simulink model "picture_prototype"  (R2022a)
settings: Solver=FixedStepAuto  StartTime=0.0  StopTime=80000  RelTol=1e-3
undefined symbols (not defined in the file): area_air, cp_air, HC_min, HC_nom, rho_air, sigbuilder_block, Ts, vel_air_nom
libraries: fl_lib x61, nesl_utility x24, SimscapeFluids_lib x5, ee_lib x4, sdl_lib x2
(part 2 of 2)

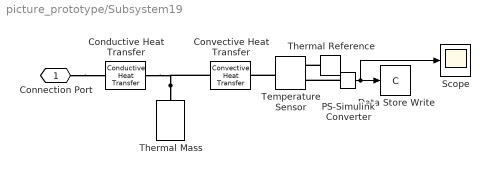
== system picture_prototype/Subsystem19 ==
  Conductive Heat Transfer : fl_lib/Thermal/Thermal Elements/Conductive Heat Transfer  area=1e-4 m^2  thickness=0.1 m  th_cond=401 W/(K*m)  T_specify=off  T_priority=None  T=0 K  T_nominal_specify=off  T_nominal_unit=K  T_nominal_value=1  Q_specify=off  Q_priority=None  Q=0 W  Q_nominal_specify=off  Q_nominal_unit=W  Q_nominal_value=1
      settings: SourceProductBaseCode=PW,SS,VE
  Convective Heat Transfer : fl_lib/Thermal/Thermal Elements/Convective Heat Transfer  area=1e-4 m^2  heat_tr_coeff=20 W/(K*m^2)  T_specify=off  T_priority=None  T=0 K  T_nominal_specify=off  T_nominal_unit=K  T_nominal_value=1  Q_specify=off  Q_priority=None  Q=0 W  Q_nominal_specify=off  Q_nominal_unit=W  Q_nominal_value=1
      settings: SourceProductBaseCode=PW,SS,VE
  Data Store Write : DataStoreWrite  DataStoreName=C  IndexOptions=Index vector (dialog)  Indices=1  OutputSizes=1
  PS-Simulink Converter : nesl_utility/PS-Simulink Converter  PhysicalDomain=network_engine_domain  SubClassName=ps_output  LeftPortType=input  RightPortType=output  PseudoPeriodic=off  Frequencies=[]  VectorFormat=inherit  Unit=inherit  AffineConversion=off
      settings: SourceProductBaseCode=SS,PW,VE
  Scope : Scope
  Temperature Sensor : fl_lib/Thermal/Thermal Sensors/Temperature Sensor
      settings: SourceProductBaseCode=PW,SS,VE
  Thermal Mass : fl_lib/Thermal/Thermal Elements/Thermal Mass  mass=1 kg  sp_heat=447 J/(K*kg)  T_specify=off  T_priority=High  T=300 K  T_nominal_specify=off  T_nominal_unit=K  T_nominal_value=1  Q_specify=off  Q_priority=None  Q=0 W  Q_nominal_specify=off  Q_nominal_unit=W  Q_nominal_value=1
      settings: SourceProductBaseCode=PW,SS,VE
  Thermal Reference : fl_lib/Thermal/Thermal Elements/Thermal Reference
      settings: SourceProductBaseCode=PW,SS,VE
  Connection Port : PMIOPort  Side=Left
  wires:
  PS-Simulink Converter/1 -> Data Store Write/1, Scope/1
  connections:
  Connection Port/RConn1 -- Conductive Heat Transfer/LConn1
  Thermal Mass/LConn1 -- Conductive Heat Transfer/RConn1 -- Convective Heat Transfer/LConn1
  Temperature Sensor/LConn1 -- Convective Heat Transfer/RConn1
  Thermal Reference/LConn1 -- Temperature Sensor/RConn1
  PS-Simulink Converter/LConn1 -- Temperature Sensor/RConn2

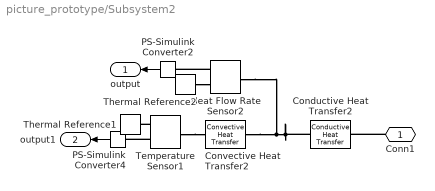
== system picture_prototype/Subsystem2 ==
  Conductive Heat Transfer2 : fl_lib/Thermal/Thermal Elements/Conductive Heat Transfer  area=1e-4 m^2  thickness=0.1 m  th_cond=401 W/(K*m)  T_specify=off  T_priority=None  T=0 K  T_nominal_specify=off  T_nominal_unit=K  T_nominal_value=1  Q_specify=off  Q_priority=None  Q=0 W  Q_nominal_specify=off  Q_nominal_unit=W  Q_nominal_value=1
      settings: SourceProductBaseCode=PW,SS,VE
  Convective Heat Transfer2 : fl_lib/Thermal/Thermal Elements/Convective Heat Transfer  area=1e-4 m^2  heat_tr_coeff=20 W/(K*m^2)  T_specify=off  T_priority=None  T=0 K  T_nominal_specify=off  T_nominal_unit=K  T_nominal_value=1  Q_specify=off  Q_priority=None  Q=0 W  Q_nominal_specify=off  Q_nominal_unit=W  Q_nominal_value=1
      settings: SourceProductBaseCode=PW,SS,VE
  Heat Flow Rate Sensor2 : fl_lib/Thermal/Thermal Sensors/Heat Flow Rate Sensor
      settings: SourceProductBaseCode=PW,SS,VE
  PS-Simulink Converter2 : nesl_utility/PS-Simulink Converter  PhysicalDomain=network_engine_domain  SubClassName=ps_output  LeftPortType=input  RightPortType=output  PseudoPeriodic=off  Frequencies=[]  VectorFormat=inherit  Unit=inherit  AffineConversion=off
      settings: SourceProductBaseCode=SS,PW,VE
  PS-Simulink Converter4 : nesl_utility/PS-Simulink Converter  PhysicalDomain=network_engine_domain  SubClassName=ps_output  LeftPortType=input  RightPortType=output  PseudoPeriodic=off  Frequencies=[]  VectorFormat=inherit  Unit=inherit  AffineConversion=off
      settings: SourceProductBaseCode=SS,PW,VE
  Temperature Sensor1 : fl_lib/Thermal/Thermal Sensors/Temperature Sensor
      settings: SourceProductBaseCode=PW,SS,VE
  Thermal Reference1 : fl_lib/Thermal/Thermal Elements/Thermal Reference
      settings: SourceProductBaseCode=PW,SS,VE
  Thermal Reference2 : fl_lib/Thermal/Thermal Elements/Thermal Reference
      settings: SourceProductBaseCode=PW,SS,VE
  Conn1 : PMIOPort  Side=Left
  output : Outport
  output1 : Outport  Port=2
  wires:
  PS-Simulink Converter2/1 -> output/1
  PS-Simulink Converter4/1 -> output1/1
  connections:
  Temperature Sensor1/RConn2 -- PS-Simulink Converter4/LConn1
  Thermal Reference2/LConn1 -- Heat Flow Rate Sensor2/RConn2
  Temperature Sensor1/RConn1 -- Thermal Reference1/LConn1
  Temperature Sensor1/LConn1 -- Convective Heat Transfer2/RConn1
  Heat Flow Rate Sensor2/RConn1 -- PS-Simulink Converter2/LConn1
  Conn1/RConn1 -- Conductive Heat Transfer2/LConn1
  Convective Heat Transfer2/LConn1 -- Conductive Heat Transfer2/RConn1 -- Heat Flow Rate Sensor2/LConn1

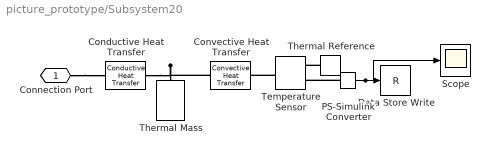
== system picture_prototype/Subsystem20 ==
  Conductive Heat Transfer : fl_lib/Thermal/Thermal Elements/Conductive Heat Transfer  area=1e-4 m^2  thickness=0.1 m  th_cond=401 W/(K*m)  T_specify=off  T_priority=None  T=0 K  T_nominal_specify=off  T_nominal_unit=K  T_nominal_value=1  Q_specify=off  Q_priority=None  Q=0 W  Q_nominal_specify=off  Q_nominal_unit=W  Q_nominal_value=1
      settings: SourceProductBaseCode=PW,SS,VE
  Convective Heat Transfer : fl_lib/Thermal/Thermal Elements/Convective Heat Transfer  area=1e-4 m^2  heat_tr_coeff=20 W/(K*m^2)  T_specify=off  T_priority=None  T=0 K  T_nominal_specify=off  T_nominal_unit=K  T_nominal_value=1  Q_specify=off  Q_priority=None  Q=0 W  Q_nominal_specify=off  Q_nominal_unit=W  Q_nominal_value=1
      settings: SourceProductBaseCode=PW,SS,VE
  Data Store Write : DataStoreWrite  DataStoreName=R  IndexOptions=Index vector (dialog)  Indices=1  OutputSizes=1
  PS-Simulink Converter : nesl_utility/PS-Simulink Converter  PhysicalDomain=network_engine_domain  SubClassName=ps_output  LeftPortType=input  RightPortType=output  PseudoPeriodic=off  Frequencies=[]  VectorFormat=inherit  Unit=inherit  AffineConversion=off
      settings: SourceProductBaseCode=SS,PW,VE
  Scope : Scope
  Temperature Sensor : fl_lib/Thermal/Thermal Sensors/Temperature Sensor
      settings: SourceProductBaseCode=PW,SS,VE
  Thermal Mass : fl_lib/Thermal/Thermal Elements/Thermal Mass  mass=1 kg  sp_heat=447 J/(K*kg)  T_specify=off  T_priority=High  T=300 K  T_nominal_specify=off  T_nominal_unit=K  T_nominal_value=1  Q_specify=off  Q_priority=None  Q=0 W  Q_nominal_specify=off  Q_nominal_unit=W  Q_nominal_value=1
      settings: SourceProductBaseCode=PW,SS,VE
  Thermal Reference : fl_lib/Thermal/Thermal Elements/Thermal Reference
      settings: SourceProductBaseCode=PW,SS,VE
  Connection Port : PMIOPort  Side=Left
  wires:
  PS-Simulink Converter/1 -> Data Store Write/1, Scope/1
  connections:
  Connection Port/RConn1 -- Conductive Heat Transfer/LConn1
  Thermal Mass/LConn1 -- Conductive Heat Transfer/RConn1 -- Convective Heat Transfer/LConn1
  Temperature Sensor/LConn1 -- Convective Heat Transfer/RConn1
  Thermal Reference/LConn1 -- Temperature Sensor/RConn1
  PS-Simulink Converter/LConn1 -- Temperature Sensor/RConn2

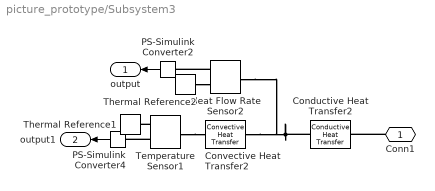
== system picture_prototype/Subsystem3 ==
  Conductive Heat Transfer2 : fl_lib/Thermal/Thermal Elements/Conductive Heat Transfer  area=1e-4 m^2  thickness=0.1 m  th_cond=401 W/(K*m)  T_specify=off  T_priority=None  T=0 K  T_nominal_specify=off  T_nominal_unit=K  T_nominal_value=1  Q_specify=off  Q_priority=None  Q=0 W  Q_nominal_specify=off  Q_nominal_unit=W  Q_nominal_value=1
      settings: SourceProductBaseCode=PW,SS,VE
  Convective Heat Transfer2 : fl_lib/Thermal/Thermal Elements/Convective Heat Transfer  area=1e-4 m^2  heat_tr_coeff=20 W/(K*m^2)  T_specify=off  T_priority=None  T=0 K  T_nominal_specify=off  T_nominal_unit=K  T_nominal_value=1  Q_specify=off  Q_priority=None  Q=0 W  Q_nominal_specify=off  Q_nominal_unit=W  Q_nominal_value=1
      settings: SourceProductBaseCode=PW,SS,VE
  Heat Flow Rate Sensor2 : fl_lib/Thermal/Thermal Sensors/Heat Flow Rate Sensor
      settings: SourceProductBaseCode=PW,SS,VE
  PS-Simulink Converter2 : nesl_utility/PS-Simulink Converter  PhysicalDomain=network_engine_domain  SubClassName=ps_output  LeftPortType=input  RightPortType=output  PseudoPeriodic=off  Frequencies=[]  VectorFormat=inherit  Unit=inherit  AffineConversion=off
      settings: SourceProductBaseCode=SS,PW,VE
  PS-Simulink Converter4 : nesl_utility/PS-Simulink Converter  PhysicalDomain=network_engine_domain  SubClassName=ps_output  LeftPortType=input  RightPortType=output  PseudoPeriodic=off  Frequencies=[]  VectorFormat=inherit  Unit=inherit  AffineConversion=off
      settings: SourceProductBaseCode=SS,PW,VE
  Temperature Sensor1 : fl_lib/Thermal/Thermal Sensors/Temperature Sensor
      settings: SourceProductBaseCode=PW,SS,VE
  Thermal Reference1 : fl_lib/Thermal/Thermal Elements/Thermal Reference
      settings: SourceProductBaseCode=PW,SS,VE
  Thermal Reference2 : fl_lib/Thermal/Thermal Elements/Thermal Reference
      settings: SourceProductBaseCode=PW,SS,VE
  Conn1 : PMIOPort  Side=Left
  output : Outport
  output1 : Outport  Port=2
  wires:
  PS-Simulink Converter2/1 -> output/1
  PS-Simulink Converter4/1 -> output1/1
  connections:
  Temperature Sensor1/RConn2 -- PS-Simulink Converter4/LConn1
  Thermal Reference2/LConn1 -- Heat Flow Rate Sensor2/RConn2
  Temperature Sensor1/RConn1 -- Thermal Reference1/LConn1
  Temperature Sensor1/LConn1 -- Convective Heat Transfer2/RConn1
  Heat Flow Rate Sensor2/RConn1 -- PS-Simulink Converter2/LConn1
  Conn1/RConn1 -- Conductive Heat Transfer2/LConn1
  Conductive Heat Transfer2/RConn1 -- Convective Heat Transfer2/LConn1 -- Heat Flow Rate Sensor2/LConn1

== system picture_prototype/fan1 ==
  Constant : Constant  Value=250
  Data Store Read : DataStoreRead  DataStoreName=T  IndexOptions=Index vector (dialog)  Indices=1  OutputSizes=1
  Fan control : Subsystem  mask(2-Level Fan Controller){T_level1=[97 94], T_level2=[105 102]}
      mask prompts: T_level1 "Level 1 temperature"; T_level2 "Level 2 temperature"
      mask help: The primary and secondary fan control temperature ranges are defined by Level 1 temperature vector and Level 2 temperature vector, respectively.
  Fan unit : Subsystem
  V_air : Outport
  wires:
  Fan control/1(U_fan) -> Fan unit/2(U_fan)
  Fan unit/1(V_air) -> V_air/1
  Constant/1 -> Fan control/1(V), Fan unit/1(Veh_speed)
  Data Store Read/1 -> Fan control/2(T)

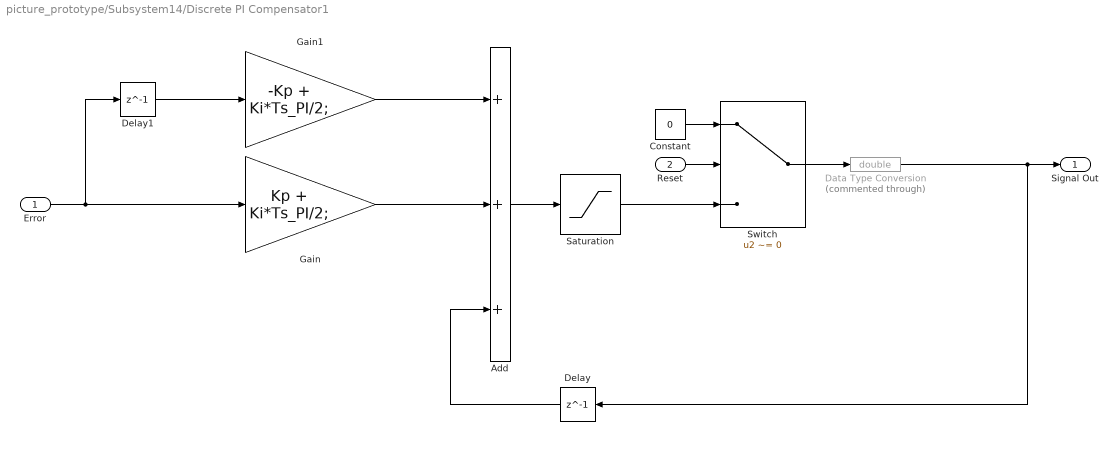
== system picture_prototype/Subsystem14/Discrete PI Compensator1 ==
  Error : Inport
  Reset : Inport  Port=2
  Add : Sum  Inputs=+++  AccumDataTypeStr=single
  Constant : Constant  Value=0
  Data Type Conversion : DataTypeConversion  Commented=through  OutDataTypeStr=double  SaturateOnIntegerOverflow=off  RndMeth=Floor
  Delay : Delay  DelayLength=1
  Delay1 : Delay  DelayLength=1  InitialCondition=Initial_Condition
  Gain : Gain  Gain=Kp + Ki*Ts_PI/2;
  Gain1 : Gain  Gain="-Kp +  Ki*Ts_PI/2;"
  Saturation : Saturate  UpperLimit=UpSat  LowerLimit=LowSat  OutDataTypeStr=single
  Switch : Switch  Criteria=u2 ~= 0  Threshold=0.5  SaturateOnIntegerOverflow=off  InputSameDT=off
  Signal Out : Outport
  wires:
  Data Type Conversion/1 -> Signal Out/1, Delay/1
  Constant/1 -> Switch/1
  Switch/1 -> Data Type Conversion/1
  Reset/1 -> Switch/2
  Saturation/1 -> Switch/3
  Gain1/1 -> Add/1
  Delay1/1 -> Gain1/1
  Gain/1 -> Add/2
  Delay/1 -> Add/3
  Error/1 -> Gain/1, Delay1/1
  Add/1 -> Saturation/1

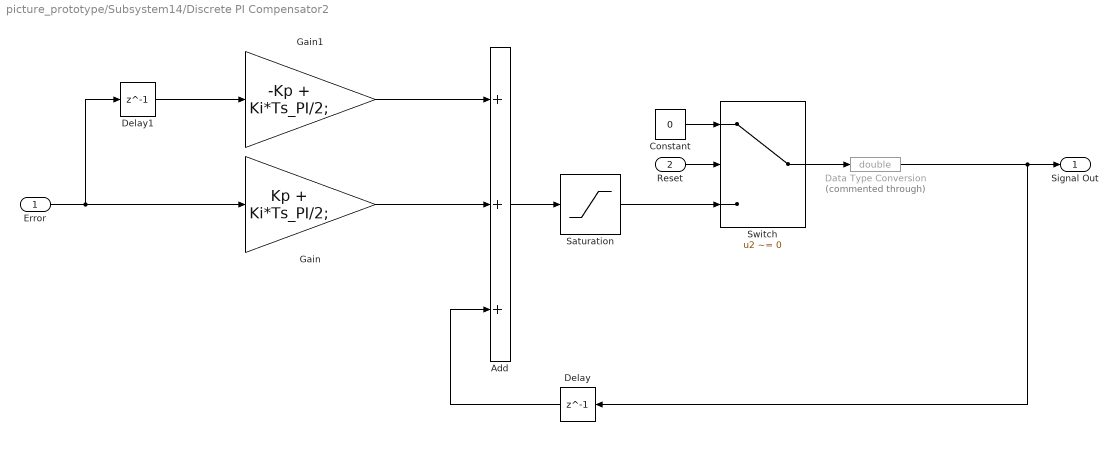
== system picture_prototype/Subsystem14/Discrete PI Compensator2 ==
  Error : Inport
  Reset : Inport  Port=2
  Add : Sum  Inputs=+++  AccumDataTypeStr=single
  Constant : Constant  Value=0
  Data Type Conversion : DataTypeConversion  Commented=through  OutDataTypeStr=double  SaturateOnIntegerOverflow=off  RndMeth=Floor
  Delay : Delay  DelayLength=1
  Delay1 : Delay  DelayLength=1  InitialCondition=Initial_Condition
  Gain : Gain  Gain=Kp + Ki*Ts_PI/2;
  Gain1 : Gain  Gain="-Kp +  Ki*Ts_PI/2;"
  Saturation : Saturate  UpperLimit=UpSat  LowerLimit=LowSat  OutDataTypeStr=single
  Switch : Switch  Criteria=u2 ~= 0  Threshold=0.5  SaturateOnIntegerOverflow=off  InputSameDT=off
  Signal Out : Outport
  wires:
  Add/1 -> Saturation/1
  Error/1 -> Delay1/1, Gain/1
  Delay/1 -> Add/3
  Gain/1 -> Add/2
  Delay1/1 -> Gain1/1
  Gain1/1 -> Add/1
  Saturation/1 -> Switch/3
  Reset/1 -> Switch/2
  Switch/1 -> Data Type Conversion/1
  Constant/1 -> Switch/1
  Data Type Conversion/1 -> Delay/1, Signal Out/1

== system picture_prototype/fan1/Fan control ==
  V : Inport
  T : Inport  Port=2
  2-level fan controller : Subsystem
  A/C com : Constant  Value=0
  K : Constant  Value=273.15
  Subtract : Sum  Inputs=+-
  To Workspace : ToWorkspace  VariableName=Fan_volt  SampleTime=-1
  U_fan : Outport  VectorParamsAs1DForOutWhenUnconnected=off
  wires:
  K/1 -> Subtract/2
  T/1 -> Subtract/1
  A/C com/1 -> 2-level fan controller/3(A/C com)
  Subtract/1 -> 2-level fan controller/2(T)
  V/1 -> 2-level fan controller/1(V)
  2-level fan controller/1(U_fan) -> To Workspace/1, U_fan/1

== system picture_prototype/fan1/Fan unit ==
  Veh_speed : Inport
  U_fan : Inport  Port=2
  2D Lookup Table : Lookup_n-D  LookupTableObject=''  BreakpointsForDimension1=[0,40,90,110,150,180,198]  BreakpointsForDimension2=[0 14.4]  Table=[0,0.8,2.2,2.7,3.6,4.1,4.6; 1.5,2.3,3.2,3.5,4.3,4.8,5.1]'  InternalRulePriority=Speed  RndMeth=Simplest
      settings: InputPortMap=u0,u1
  Scope : Scope  NumInputPorts=3
  Transfer Fcn : TransferFcn  Denominator=[10 1]
  V_air : Outport  VectorParamsAs1DForOutWhenUnconnected=off
  wires:
  Veh_speed/1 -> Scope/2, 2D Lookup Table/1  "Veh_speed"
  2D Lookup Table/1 -> Transfer Fcn/1
  U_fan/1 -> Scope/3, 2D Lookup Table/2  "U_fan"
  Transfer Fcn/1 -> Scope/1, V_air/1  "V_air"

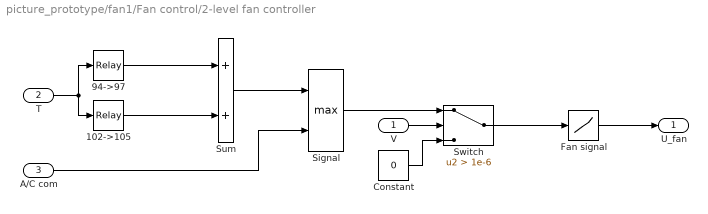
== system picture_prototype/fan1/Fan control/2-level fan controller ==
  V : Inport
  T : Inport  Port=2
  A/C com : Inport  Port=3
  102->105 : Relay  OnSwitchValue=T_level2(1)  OffSwitchValue=T_level2(2)
  94->97 : Relay  OnSwitchValue=T_level1(1)  OffSwitchValue=T_level1(2)
  Constant : Constant  Value=0
  Fan signal : Lookup  InputValues=[0, 1, 2]  Table=[0, 5, 14.4]
  Signal : MinMax  Function=max  Inputs=2  InputSameDT=on  SaturateOnIntegerOverflow=on
  Sum : Sum  Inputs=2  InputSameDT=on  SaturateOnIntegerOverflow=on  OutDataTypeStr=Inherit: Same as first input
  Switch : Switch  Criteria=u2 > Threshold  Threshold=1e-6  ZeroCross=off  SaturateOnIntegerOverflow=off  InputSameDT=off
  U_fan : Outport  VectorParamsAs1DForOutWhenUnconnected=off
  wires:
  Fan signal/1 -> U_fan/1
  T/1 -> 102->105/1, 94->97/1
  102->105/1 -> Sum/2
  94->97/1 -> Sum/1
  Sum/1 -> Signal/1
  Signal/1 -> Switch/1
  A/C com/1 -> Signal/2
  V/1 -> Switch/2
  Constant/1 -> Switch/3
  Switch/1 -> Fan signal/1
